simulink model "AxleSplitHEVv6"  (Simulink 8.5)
settings: Solver=ode5  StartTime=0.0  StopTime=hev_te  FixedStep=hev_dt  MaxStep=0.01  RelTol=1e-3  AbsTol=1e-3
PostLoadFcn:
  | load('AxelSplitHEVv4_NEDC_18_06_15.mat')
values from neighbouring files (symbols this model uses):
  cmd_equivalent_conso_coef = 0.11126984    [AxelSplitHEVv4_NEDC_18_06_15.mat]
  cmd_qmax = 42    [AxelSplitHEVv4_NEDC_18_06_15.mat]
  cmd_specific_volume_l_per_g = 0.00133333333333    [AxelSplitHEVv4_NEDC_18_06_15.mat]
  dri_cycle_speed_sp = [0 0 0 4.16666667 4.16666667 2.777777778 0 0 0 4.166666667 4.166666667 8.88888889 ... (135 elements, 135x1)]    [AxelSplitHEVv4_NEDC_18_06_15.mat]
  dri_cycle_speed_time = [0 6 11 15 23 25 28 44 49 54 56 61 ... (135 elements, 135x1)]    [AxelSplitHEVv4_NEDC_18_06_15.mat]
  dri_gbx_sp = [0 1 0 1 2 0 1 2 3 2 0 1 ... (52 elements, 52x1)]    [AxelSplitHEVv4_NEDC_18_06_15.mat]
  dri_gbx_time = [0 11 25 49 55 93 117 123 134 177 185 206 ... (52 elements, 52x1)]    [AxelSplitHEVv4_NEDC_18_06_15.mat]
  dri_ki = 24.5    [AxelSplitHEVv4_NEDC_18_06_15.mat]
  dri_kp = 609    [AxelSplitHEVv4_NEDC_18_06_15.mat]
  fa_clu_pos = [1 1 0.7 0.5 0.3 0 0]    [AxelSplitHEVv4_NEDC_18_06_15.mat]
  fa_clu_pv = [0 0.1 0.3 0.5 0.7 0.9 1]    [AxelSplitHEVv4_NEDC_18_06_15.mat]
  fa_conso_idle = 0.153611111111    [AxelSplitHEVv4_NEDC_18_06_15.mat]
  fa_conso_speed = [200 300 400 500 600 700 800 900 1000 1100 1200 1300 ... (56 elements, 1x56)]    [AxelSplitHEVv4_NEDC_18_06_15.mat]
  fa_conso_torque = [0 6.66666666667 13.3333333333 20 26.6666666667 33.3333333333 40 46.6666666667 53.3333333333 60 66.6666666667 73.3333333333 ... (43 elements, 1x43)]    [AxelSplitHEVv4_NEDC_18_06_15.mat]
  fa_delta_derating = 500    [AxelSplitHEVv4_NEDC_18_06_15.mat]
  fa_differential_ratio = FDR.fa_differential_ratio    [Algorithme_eff.m]    (also in AxelSplitHEVv4_NEDC_18_06_15.mat = 3.72; fa_differential_ratio.mat = 3.72)
  fa_fuel_consumption = [nan nan nan nan nan nan nan nan nan nan nan nan ... (2408 elements, 43x56)]    [AxelSplitHEVv4_NEDC_18_06_15.mat]    (also in Curve_fitting_conso.m = fa_fuel_consumption/max(max(fa_fuel_consumption)))
  fa_gearbox_efficiency = 0.92    [AxelSplitHEVv4_NEDC_18_06_15.mat]
  fa_gearbox_ratio = FGR.fa_gearbox_ratio    [Algorithme_eff.m]    (also in AxelSplitHEVv4_NEDC_18_06_15.mat = [0 3.98 2.21 1.47 1.1 0.89 0.75]; fa_gearbox_ratio.mat = [0 3.98 2.21 1.47 1.1 0.89 0.75])
  fa_high_derating_point = 5700    [AxelSplitHEVv4_NEDC_18_06_15.mat]
  fa_ice_inertia = 0.058    [AxelSplitHEVv4_NEDC_18_06_15.mat]
  fa_kp_idle_tr_off = 0.116198282851    [AxelSplitHEVv4_NEDC_18_06_15.mat]
  fa_kp_idle_tr_on = [1 0.8653 2.8063 6.3428 11.3274 17.3036 24.3665]    [AxelSplitHEVv4_NEDC_18_06_15.mat]
  fa_low_derating_point = 4000    [AxelSplitHEVv4_NEDC_18_06_15.mat]
  fa_max_tq_clu = 206    [AxelSplitHEVv4_NEDC_18_06_15.mat]
  fa_max_tq_ice = [0 220 233.333333333 240 246.666666667 253.333333333 253.333333333 253.333333333 260 260 266.666666667 266.666666667 ... (52 elements, 1x52)]    [AxelSplitHEVv4_NEDC_18_06_15.mat]
  fa_n_ice = [0 20 250 850 1000 1250 1500 1750 2000 2250 2500 3000 ... (18 elements, 1x18)]    [AxelSplitHEVv4_NEDC_18_06_15.mat]
  fa_starter_rpm = [0 10 20 30 40 50 60 70 80 90 100 110 ... (101 elements, 1x101)]    [AxelSplitHEVv4_NEDC_18_06_15.mat]
  fa_starter_tq = [24 24 24 24 23.3333333333 23.3333333333 23.3333333333 22.6666666667 22.6666666667 22 21.3333333333 20.6666666667 ... (101 elements, 1x101)]    [AxelSplitHEVv4_NEDC_18_06_15.mat]
  fa_tau_ice = 0.0333    [AxelSplitHEVv4_NEDC_18_06_15.mat]
  fa_taui_idle_tr_off = 0.0820482966067    [AxelSplitHEVv4_NEDC_18_06_15.mat]
  fa_taui_idle_tr_on = 0.194086623254    [AxelSplitHEVv4_NEDC_18_06_15.mat]
  fa_tq_loss = [0 -11 -10 -9 -9 -10 -11 -11 -12 -13 -14 -15 ... (18 elements, 1x18)]    [AxelSplitHEVv4_NEDC_18_06_15.mat]
  fa_tq_max_speed = [200 700 800 900 1000 1100 1200 1300 1400 1500 1600 1700 ... (52 elements, 1x52)]    [AxelSplitHEVv4_NEDC_18_06_15.mat]
  hev_dt = 0.01    [AxelSplitHEVv4_NEDC_18_06_15.mat]
  pla_csat = 1.2    [AxelSplitHEVv4_NEDC_18_06_15.mat]
  pla_equivalent_weight = 1250    [AxelSplitHEVv4_NEDC_18_06_15.mat]
  pla_f = 0.0035272    [AxelSplitHEVv4_NEDC_18_06_15.mat]
  pla_k = 0.0002318    [AxelSplitHEVv4_NEDC_18_06_15.mat]
  pla_kaero = 0.52992    [AxelSplitHEVv4_NEDC_18_06_15.mat]
  pla_max_f_brakes = 1000    [AxelSplitHEVv4_NEDC_18_06_15.mat]
  pla_wheel_radius = 0.314    [AxelSplitHEVv4_NEDC_18_06_15.mat]
  ra_differential_ratio = RDR.ra_differential_ratio    [Algorithme_eff.m]    (also in AxelSplitHEVv4_NEDC_18_06_15.mat = 10; ra_differential_ratio.mat = 10)
  ra_electrical_machine_efficiency = [nan nan nan nan nan nan nan 91.3 91.3 91.3 91.5 91.3 ... (777 elements, 37x21)]    [AxelSplitHEVv4_NEDC_18_06_15.mat]
  ra_electrical_machine_speed = [-12000 -10800 -9600 -8400 -7200 -6000 -4800 -3600 -2400 -1200 0 1200 ... (21 elements, 1x21)]    [AxelSplitHEVv4_NEDC_18_06_15.mat]
  ra_electrical_machine_tau = 0.1    [AxelSplitHEVv4_NEDC_18_06_15.mat]
  ra_electrical_machine_torque = [-79.6460176991 -75.2212389381 -70.796460177 -66.3716814159 -61.9469026549 -57.5221238938 -53.0973451327 -48.6725663717 -44.2477876106 -39.8230088496 -35.3982300885 -30.9734513274 ... (37 elements, 1x37)]    [AxelSplitHEVv4_NEDC_18_06_15.mat]
  ra_em_max_tq = [39.8230088496 44.2477876106 53.0973451327 57.5221238938 70.796460177 79.6460176991 79.6460176991 79.6460176991 79.6460176991 79.6460176991 79.6460176991 79.6460176991 ... (21 elements, 1x21)]    [AxelSplitHEVv4_NEDC_18_06_15.mat]
  ra_em_min_tq = [-39.8230088496 -44.2477876106 -53.0973451327 -57.5221238938 -70.796460177 -79.6460176991 -79.6460176991 -79.6460176991 -79.6460176991 -79.6460176991 -79.6460176991 -79.6460176991 ... (21 elements, 1x21)]    [AxelSplitHEVv4_NEDC_18_06_15.mat]
  ra_transmission_efficiency = 0.92    [AxelSplitHEVv4_NEDC_18_06_15.mat]
  syse_aux_current = 33.3    [AxelSplitHEVv4_NEDC_18_06_15.mat]
  syse_aux_voltage = 12    [AxelSplitHEVv4_NEDC_18_06_15.mat]
  syse_bat_nominal_capacity_as = 151200    [AxelSplitHEVv4_NEDC_18_06_15.mat]
  syse_cdl = 5000    [AxelSplitHEVv4_NEDC_18_06_15.mat]
  syse_dcdc_efficency = [78 89.6 92.5 95.2 95 94.6]    [AxelSplitHEVv4_NEDC_18_06_15.mat]
  syse_dcdc_in_power = [54 135 202 405 1485 2000]    [AxelSplitHEVv4_NEDC_18_06_15.mat]
  syse_electrical_machine_torque_vs_power_speed_nneg = [38.4209635438 42.3166718474 53.0973451327 53.8788373627 63.500986907 77.9700595469 78.3175021924 76.9635177026 72.2987813984 47.9837613501 38.4209635438 42.3166718474 ... (220 elements, 10x22)]    [AxelSplitHEVv4_NEDC_18_06_15.mat]
  syse_electrical_machine_torque_vs_power_speed_npos = [-72.2987813984 -76.9635177026 -78.3175021924 -77.9700595469 -63.500986907 -53.8788373627 -53.0973451327 -42.3166718474 -38.4209635438 -72.2987813984 -76.9635177026 -78.3175021924 ... (198 elements, 9x22)]    [AxelSplitHEVv4_NEDC_18_06_15.mat]
  syse_em_in_power = [-49.1089315336 -44.1089315336 -39.1089315336 -34.1089315336 -29.1089315336 -24.1089315336 -19.1089315336 -14.1089315336 -9.10893153364 -4.10893153364 0.891068466363 5.89106846636 ... (22 elements, 1x22)]    [AxelSplitHEVv4_NEDC_18_06_15.mat]
  syse_max_charge_current = [8.4 8.4 42 92.4 92.4 92.4 92.4 92.4 79.8 42 21 4.2]    [AxelSplitHEVv4_NEDC_18_06_15.mat]
  syse_max_discharge_current = [42 42 79.8 159.6 180.6 180.6 180.6 180.6 180.6 180.6 180.6 180.6]    [AxelSplitHEVv4_NEDC_18_06_15.mat]
  syse_nb_cell = 52    [AxelSplitHEVv4_NEDC_18_06_15.mat]
  syse_rdl = 0.004    [AxelSplitHEVv4_NEDC_18_06_15.mat]
  syse_rser = 0.002    [AxelSplitHEVv4_NEDC_18_06_15.mat]
  syse_soc_current_limits = [0 10 20 20.1 30 40 50 60 70 80 90 100]    [AxelSplitHEVv4_NEDC_18_06_15.mat]
  syse_soc_initial = 0.8    [AxelSplitHEVv4_NEDC_18_06_15.mat]
  syse_soc_ocv = [0 5 10 20 40 50 60 70 80 90 100]    [AxelSplitHEVv4_NEDC_18_06_15.mat]
  syse_vocv = [2.5 3.2135 3.5127 3.66 3.7771 3.8181 3.8686 3.8978 3.9429 4.0006 4.198]    [AxelSplitHEVv4_NEDC_18_06_15.mat]
libraries: simulink x20, simulink_extras x1
(part 2 of 3)

== system AxleSplitHEVv6/HEV model/Command/Braking_repartition/BREAKE REPARTITION RA ==
  CMD_RA_BREAK : Inport
  SYSE_SOC : Inport  Port=2
  RA_TQ_MIN : Inport  Port=3
  Add : Sum  Inputs=+-
  Add1 : Sum  Inputs=++|
  Add2 : Sum  Inputs=|+-
  Constant : Constant  Tag=Soc_level  Value=0.9
  Gain : Gain  Gain=-1
  Ground : Ground
  Switch : Switch  Criteria=u2 > Threshold
  Switch1 : Switch  Criteria=u2 > Threshold
  CMD_RA_MECHANICAL_BRAKE : Outport
  CMD_RA_ELECTRICAL_BRAKE : Outport  Port=2
  wires:
  CMD_RA_BREAK/1 -> Add1/1, Switch1/3, Add2/1
  Switch1/1 -> CMD_RA_ELECTRICAL_BRAKE/1, Add2/2
  Add1/1 -> Switch1/2
  Ground/1 -> Switch/1
  RA_TQ_MIN/1 -> Switch/3
  Switch/1 -> Gain/1, Add1/2
  Add2/1 -> CMD_RA_MECHANICAL_BRAKE/1
  SYSE_SOC/1 -> Add/1
  Constant/1 -> Add/2
  Add/1 -> Switch/2
  Gain/1 -> Switch1/1

== system AxleSplitHEVv6/HEV model/Command/Start_Stop/startstop prototype ==
  PLA_N : Inport
  DRI_GBX_SP : Inport  Port=2
  START_STOP_ENABLE : Inport  Port=3
  DRI_CLUTCH_SP : Inport  Port=4
  Activate Start/Stopo strategy : Constant  Value=0
  Logical Operator1 : Logic  Inputs=3  AllPortsSameDT=off  OutDataTypeStr=boolean  SampleTime=hev_dt
  Switch : Switch  Criteria=u2 ~= 0  SampleTime=hev_dt
  car_moving : simulink/Logic and Bit Operations/Compare To Constant  relop=<=  const=0.04  OutDataTypeStr=uint8
  clutch_pedal_down : simulink/Logic and Bit Operations/Compare To Constant  relop===  const=1  OutDataTypeStr=uint8
  gbx_not_neutral : simulink/Logic and Bit Operations/Compare To Constant  relop===  const=0  OutDataTypeStr=uint8
  CMD_ICE_ENABLE : Outport
  wires:
  PLA_N/1 -> car_moving/1
  car_moving/1 -> Logical Operator1/1
  gbx_not_neutral/1 -> Logical Operator1/3
  Activate Start/Stopo strategy/1 -> Switch/3
  Logical Operator1/1 -> Switch/1
  DRI_GBX_SP/1 -> gbx_not_neutral/1
  START_STOP_ENABLE/1 -> Switch/2
  Switch/1 -> CMD_ICE_ENABLE/1
  DRI_CLUTCH_SP/1 -> clutch_pedal_down/1
  clutch_pedal_down/1 -> Logical Operator1/2

== system AxleSplitHEVv6/HEV model/Command/Torque repartition/Optimization Algorithm  ==
  note: Filtrage du alpha
  T : Inport
  PLA_N : Inport  Port=2
  Tmax_elec : Inport  Port=3
  Tmin_elec : Inport  Port=4
  Tmax_therm : Inport  Port=5
  Tmin_therm : Inport  Port=6
  DRI_GBX : Inport  Port=7
  "SOC " : Inport  Port=8
  Doc Front axle : Subsystem
      settings: OpenFcn=open('Documents\Command Torque Repartition Algorithm.pdf')
      mask Display: fprintf('DOC')
  Doc Front axle1 : Subsystem
      settings: OpenFcn=open('Optimization_Algorithm')
      mask Display: fprintf('Generate\nOptimization\nAlgorithm\nSfunction')
  Sfunction: Optimization Algorithm 32bits : Subsystem
      mask help: Simulink:masks:GenSFuncDesc_MD
      mask Help: eval('feval(''rtwprivate'',''rtwhelpview'',''rtw_sfcn_block'')');
  Transfer Fcn : TransferFcn  Denominator=[1 3/2]
  alpha : Outport
  wires:
  Tmax_elec/1 -> Sfunction: Optimization Algorithm 32bits/3(Tmax_elec)
  Tmin_elec/1 -> Sfunction: Optimization Algorithm 32bits/4(Tmin_elec)
  PLA_N/1 -> Sfunction: Optimization Algorithm 32bits/2(V)
  Tmax_therm/1 -> Sfunction: Optimization Algorithm 32bits/5(Tmax_therm)
  T/1 -> Sfunction: Optimization Algorithm 32bits/1(T)
  Tmin_therm/1 -> Sfunction: Optimization Algorithm 32bits/6(Tmin_therm)
  DRI_GBX/1 -> Sfunction: Optimization Algorithm 32bits/7(GBX)
  "SOC "/1 -> Sfunction: Optimization Algorithm 32bits/8(SOC)
  Transfer Fcn/1 -> alpha/1
  Sfunction: Optimization Algorithm 32bits/1(alpha_opt) -> Transfer Fcn/1

== system AxleSplitHEVv6/HEV model/Command/Torque repartition/energy_manager Stop thermal engine when <20km/h ==
  note: Energy managment modified : Not taking account of the FA_START command
      | Cf. Previous model
  PLA_N : Inport
  alpha_in : Inport  Port=2
  SOC : Inport  Port=3
  Compare To Constant : simulink/Logic and Bit Operations/Compare To Constant  relop=<  const=20  OutDataTypeStr=boolean
  Compare To Constant1 : simulink/Logic and Bit Operations/Compare To Constant  relop=>  const=0.2  OutDataTypeStr=boolean
  Constant3 : Constant  Value=0
  Gain : Gain  Gain=(60*(2*pi*pla_wheel_radius))/1e3
  Logical Operator1 : Logic  AllPortsSameDT=off  OutDataTypeStr=boolean
  Switch : Switch  Criteria=u2 > Threshold
  alpha_out : Outport
  CMD_ENERGY_MANAGER : Outport  Port=2
  wires:
  SOC/1 -> Compare To Constant1/1
  PLA_N/1 -> Gain/1
  Logical Operator1/1 -> CMD_ENERGY_MANAGER/1, Switch/2
  Compare To Constant1/1 -> Logical Operator1/1
  Gain/1 -> Compare To Constant/1
  Constant3/1 -> Switch/1
  alpha_in/1 -> Switch/3
  Switch/1 -> alpha_out/1
  Compare To Constant/1 -> Logical Operator1/2

== system AxleSplitHEVv6/HEV model/Driver1/Clutch command/Clutch Command ==
  note: SHIFT DOWN
  note: SHIFT UP
  DRI_REF_GBX : Inport
  Data Type Conversion : DataTypeConversion  OutDataTypeStr=double
  Data Type Conversion1 : DataTypeConversion  OutDataTypeStr=double
  Delay : Delay  DelayLength=1/hev_dt
  Delay1 : Delay  DelayLength=1
  Delay2 : Delay  DelayLength=1
  SHIFT DOWN : Stateflow chart  TreatAsAtomicUnit=on
  SHIFT UP : Stateflow chart  TreatAsAtomicUnit=on
  Sum2 : Sum
  To Workspace : ToWorkspace  VariableName=GBX_reference  SampleTime=-1
  Transfer Fcn{1..4} (4 alike) : TransferFcn  Denominator=[0.1 1]
  DRI_CLUTCH_SP : Outport
  DRI_GBX_SP : Outport  Port=2
  wires:
  SHIFT UP/1(output_memory) -> Data Type Conversion/1
  Sum2/1 -> DRI_CLUTCH_SP/1
  SHIFT DOWN/1(output_memory) -> Data Type Conversion1/1
  Delay2/1 -> SHIFT DOWN/1(last_DRI_REF_GBX)
  DRI_REF_GBX/1 -> SHIFT UP/2(DRI_REF_GBX), Delay1/1, Delay/1, SHIFT DOWN/2(DRI_REF_GBX), Delay2/1, To Workspace/1
  Delay/1 -> SHIFT UP/3(actual_DRI_GBX), DRI_GBX_SP/1, SHIFT DOWN/3(actual_DRI_GBX)
  Delay1/1 -> SHIFT UP/1(last_DRI_REF_GBX)
  Transfer Fcn1/1 -> Transfer Fcn2/1
  Data Type Conversion/1 -> Transfer Fcn1/1
  Transfer Fcn3/1 -> Transfer Fcn4/1
  Data Type Conversion1/1 -> Transfer Fcn3/1
  Transfer Fcn2/1 -> Sum2/1
  Transfer Fcn4/1 -> Sum2/2

== system AxleSplitHEVv6/HEV model/Driver1/Clutch command/Clutch Stuck ==
  REF_GBX : Inport
  FA_N_ICE : Inport  Port=2
  DRI_CLU_SP : Inport  Port=3
  1/time pedal down->up  gbx 1st gear : Constant  Value=-1/2
  1/time pedal up->down : Constant  Value=2
  Compare To Constant : simulink/Logic and Bit Operations/Compare To Constant  relop=>=  const=2000  OutDataTypeStr=boolean
  Compare To Constant1 : simulink/Logic and Bit Operations/Compare To Constant  relop=<  const=800  OutDataTypeStr=boolean
  Compare To Constant3 : simulink/Logic and Bit Operations/Compare To Constant  relop===  const=0  OutDataTypeStr=uint8
  Compare To Constant4 : simulink/Logic and Bit Operations/Compare To Constant  relop=~=  const=0  OutDataTypeStr=uint8
  Data Type Conversion4 : DataTypeConversion  OutDataTypeStr=double  SampleTime=hev_dt
  Delay1 : Delay  DelayLength=2/hev_dt  SampleTime=hev_dt
  Delay2 : Delay  DelayLength=1  SampleTime=hev_dt
  Logical Operator1 : Logic  Operator=OR  AllPortsSameDT=off  OutDataTypeStr=boolean  SampleTime=hev_dt
  Logical Operator7 : Logic  Inputs=3  AllPortsSameDT=off  OutDataTypeStr=boolean  SampleTime=hev_dt
  Rate Limiter Dynamic : simulink/Discontinuities/Rate Limiter Dynamic
  S-R Flip-Flop : simulink_extras/Flip Flops/S-R Flip-Flop  initial_condition=0
  Switch : Switch  Criteria=u2 > Threshold
  Terminator : Terminator
  OUT_CLU : Outport
  wires:
  REF_GBX/1 -> Delay2/1, Compare To Constant4/1
  S-R Flip-Flop/2 -> Terminator/1
  Compare To Constant/1 -> S-R Flip-Flop/2
  Rate Limiter Dynamic/1 -> Switch/1
  S-R Flip-Flop/1 -> Logical Operator1/2, Delay1/1, Data Type Conversion4/1
  Compare To Constant4/1 -> Logical Operator7/1
  Delay2/1 -> Compare To Constant3/1
  Compare To Constant3/1 -> Logical Operator7/2
  FA_N_ICE/1 -> Compare To Constant/1, Compare To Constant1/1
  Delay1/1 -> Logical Operator1/1
  Data Type Conversion4/1 -> Rate Limiter Dynamic/2
  1/time pedal up->down/1 -> Rate Limiter Dynamic/1
  Compare To Constant1/1 -> Logical Operator7/3
  Logical Operator1/1 -> Switch/2
  Logical Operator7/1 -> S-R Flip-Flop/1
  1/time pedal down->up  gbx 1st gear/1 -> Rate Limiter Dynamic/3
  Switch/1 -> OUT_CLU/1
  DRI_CLU_SP/1 -> Switch/3

== system AxleSplitHEVv6/HEV model/Electrical system/Auxiliary network 12V/Auxliliary network ==
  Constant : Constant  Value=syse_aux_current
  Constant1 : Constant  Value=syse_aux_voltage
  SYSE_CURRENT_LV : Outport
  SYSE_VOLTAGE_LV : Outport  Port=2
  wires:
  Constant/1 -> SYSE_CURRENT_LV/1  "A"
  Constant1/1 -> SYSE_VOLTAGE_LV/1  "V"

== system AxleSplitHEVv6/HEV model/Electrical system/Auxiliary network 12V/CVS ==
  note: V
  SYSE_CURRENT_LV : Inport
  SYSE_VOLTAGE_LV : Inport  Port=2
  SYSE_VOLTAGE_HV : Inport  Port=3
  Delay : Delay  DelayLength=1  SampleTime=hev_dt
  Divide : Product  Inputs=/*  SampleTime=hev_dt
  Divide1 : Product  Inputs=*/  SampleTime=hev_dt
  Product : Product  SampleTime=hev_dt  RndMeth=Zero
  rendement CVS : Lookup_n-D  NumberOfTableDimensions=1  BreakpointsForDimension1=syse_dcdc_in_power.*(syse_dcdc_efficency/100)  Table=syse_dcdc_efficency/100  SampleTime=hev_dt  RndMeth=Simplest  InputSameDT=on
  SYSE_AUX_CURRENT : Outport
  wires:
  rendement CVS/1 -> Divide/1
  Divide/1 -> Divide1/1  "W"
  Product/1 -> Divide/2, rendement CVS/1  "W"
  SYSE_VOLTAGE_HV/1 -> Divide1/2
  SYSE_CURRENT_LV/1 -> Product/1
  SYSE_VOLTAGE_LV/1 -> Product/2
  Divide1/1 -> Delay/1
  Delay/1 -> SYSE_AUX_CURRENT/1

== system AxleSplitHEVv6/HEV model/Electrical system/Electrical System supervision/Battery charge / discharge limits ==
  SYSE_SOC : Inport
  Courant Charge Lookup Table : Lookup_n-D  NumberOfTableDimensions=1  BreakpointsForDimension1=syse_soc_current_limits/100  Table=-syse_max_charge_current  SampleTime=hev_dt  RndMeth=Simplest  InputSameDT=on
  Courant Decharge Lookup Table : Lookup_n-D  NumberOfTableDimensions=1  BreakpointsForDimension1=syse_soc_current_limits/100  Table=syse_max_discharge_current  SampleTime=hev_dt  RndMeth=Simplest  InputSameDT=on
  SYSE_I_DISCHARGE : Outport
  SYSE_I_CHARGE : Outport  Port=2
  wires:
  SYSE_SOC/1 -> Courant Decharge Lookup Table/1, Courant Charge Lookup Table/1
  Courant Decharge Lookup Table/1 -> SYSE_I_DISCHARGE/1
  Courant Charge Lookup Table/1 -> SYSE_I_CHARGE/1

== system AxleSplitHEVv6/HEV model/Electrical system/Electrical System supervision/Current loop ==
  SYSE_AUX_CURRENT : Inport
  SYSE_I_DISCHARGE : Inport  Port=2
  SYSE_I_CHARGE : Inport  Port=3
  Subtract2 : Sum  Inputs=-+  SampleTime=hev_dt
  Subtract3 : Sum  SampleTime=hev_dt
  SYSE_EM_I_DISCHARGE : Outport
  SYSE_EM_I_CHARGE : Outport  Port=2
  wires:
  SYSE_AUX_CURRENT/1 -> Subtract2/1, Subtract3/1  "A"
  Subtract2/1 -> SYSE_EM_I_DISCHARGE/1  "A"
  SYSE_I_DISCHARGE/1 -> Subtract2/2  "A"
  Subtract3/1 -> SYSE_EM_I_CHARGE/1  "A"
  SYSE_I_CHARGE/1 -> Subtract3/2  "A"

== system AxleSplitHEVv6/HEV model/Electrical system/Electrical System supervision/Min max  ==
  note: RPM
  SYSE_EM_I_DISCHARGE : Inport
  SYSE_EM_I_CHARGE : Inport  Port=2
  SYSE_VOLTAGE_HV : Inport  Port=3
  PLA_N_EM : Inport  Port=4
  Min /w power neg : Lookup_n-D  BreakpointsForDimension1=ra_electrical_machine_speed(1:10)  BreakpointsForDimension2=syse_em_in_power*1000  Table=syse_electrical_machine_torque_vs_power_speed_nneg  ExtrapMethod=Clip  UseLastTableValue=on  SampleTime=hev_dt  RndMeth=Simplest  InputSameDT=on
  Min /w power pos : Lookup_n-D  BreakpointsForDimension1=ra_electrical_machine_speed(12:20)  BreakpointsForDimension2=syse_em_in_power*1000  Table=syse_electrical_machine_torque_vs_power_speed_npos  ExtrapMethod=Clip  UseLastTableValue=on  SampleTime=hev_dt  RndMeth=Simplest  InputSameDT=on
  Product : Product  SampleTime=hev_dt  RndMeth=Zero
  Product2 : Product  SampleTime=hev_dt  RndMeth=Zero
  Switch : Switch  Threshold=-5  SampleTime=hev_dt
  Switch1 : Switch  Threshold=-5  SampleTime=hev_dt
  max /w power neg : Lookup_n-D  BreakpointsForDimension1=ra_electrical_machine_speed(1:10)  BreakpointsForDimension2=syse_em_in_power*1000  Table=syse_electrical_machine_torque_vs_power_speed_nneg  ExtrapMethod=Clip  UseLastTableValue=on  SampleTime=hev_dt  RndMeth=Simplest  InputSameDT=on
  max /w power pos : Lookup_n-D  BreakpointsForDimension1=ra_electrical_machine_speed(12:20)  BreakpointsForDimension2=syse_em_in_power*1000  Table=syse_electrical_machine_torque_vs_power_speed_npos  ExtrapMethod=Clip  UseLastTableValue=on  SampleTime=hev_dt  RndMeth=Simplest  InputSameDT=on
  SYSE_TQ_MAX_BMS : Outport
  SYSE_TQ_MIN_BMS : Outport  Port=2
  wires:
  PLA_N_EM/1 -> Min /w power pos/1, Min /w power neg/1, Switch1/2, max /w power pos/1, max /w power neg/1, Switch/2
  SYSE_EM_I_DISCHARGE/1 -> Product/1  "A"
  SYSE_EM_I_CHARGE/1 -> Product2/1  "A"
  Product2/1 -> Min /w power pos/2, Min /w power neg/2  "W"
  Product/1 -> max /w power neg/2, max /w power pos/2  "W"
  SYSE_VOLTAGE_HV/1 -> Product2/2, Product/2
  Switch/1 -> SYSE_TQ_MAX_BMS/1
  max /w power pos/1 -> Switch/1
  max /w power neg/1 -> Switch/3  "Nm"
  Min /w power pos/1 -> Switch1/1  "Nm"
  Min /w power neg/1 -> Switch1/3
  Switch1/1 -> SYSE_TQ_MIN_BMS/1

== system AxleSplitHEVv6/HEV model/Electrical system/Electrical System supervision/Torque conversion ==
  SYSE_TQ_MINMAX_BMS : Inport
  RA_N_EM : Inport  Port=2
  Differential ratio : Gain  Gain=ra_differential_ratio  SampleTime=hev_dt
  Divide1 : Product  SampleTime=hev_dt
  Efficiency P neg : Gain  Gain=2-ra_transmission_efficiency  SampleTime=hev_dt
  Efficiency P pos : Gain  Gain=ra_transmission_efficiency  SampleTime=hev_dt
  Switch : Switch  SampleTime=hev_dt
  SYSE_TQ_MINMAX : Outport
  wires:
  SYSE_TQ_MINMAX_BMS/1 -> Divide1/2, Efficiency P neg/1, Efficiency P pos/1
  Efficiency P pos/1 -> Switch/1
  Efficiency P neg/1 -> Switch/3
  Divide1/1 -> Switch/2
  Switch/1 -> Differential ratio/1
  RA_N_EM/1 -> Divide1/1
  Differential ratio/1 -> SYSE_TQ_MINMAX/1

== system AxleSplitHEVv6/HEV model/Electrical system/Lithium-Ion Battery Management System/Battery control ==
  note: Battery safety system
  SYSE_LIION_CURRENT : Inport
  SYSE_SOC : Inport  Port=2
  Courant Charge Lookup Table : Lookup_n-D  NumberOfTableDimensions=1  BreakpointsForDimension1=syse_soc_current_limits/100  Table=-syse_max_charge_current  SampleTime=hev_dt  RndMeth=Simplest  InputSameDT=on
  Courant Decharge Lookup Table : Lookup_n-D  NumberOfTableDimensions=1  BreakpointsForDimension1=syse_soc_current_limits/100  Table=syse_max_discharge_current  SampleTime=hev_dt  RndMeth=Simplest  InputSameDT=on
  Logical Operator : Logic  AllPortsSameDT=off  OutDataTypeStr=boolean  SampleTime=hev_dt
  Relational Operator : RelationalOperator  Operator=<  OutDataTypeStr=boolean  SampleTime=hev_dt
  Relational Operator1 : RelationalOperator  Operator=>  OutDataTypeStr=boolean  SampleTime=hev_dt
  SYSE_LIION_CONTACTOR_OPEN_REQ : Outport
  wires:
  SYSE_LIION_CURRENT/1 -> Relational Operator/1, Relational Operator1/1  "A"
  Courant Charge Lookup Table/1 -> Relational Operator/2  "syse_max_charge_current (A)"
  Courant Decharge Lookup Table/1 -> Relational Operator1/2  "syse_max_discharge_current (A)"
  SYSE_SOC/1 -> Courant Charge Lookup Table/1, Courant Decharge Lookup Table/1
  Logical Operator/1 -> SYSE_LIION_CONTACTOR_OPEN_REQ/1
  Relational Operator/1 -> Logical Operator/1
  Relational Operator1/1 -> Logical Operator/2

== system AxleSplitHEVv6/HEV model/Electrical system/Lithium-Ion Battery Management System/Battery model ==
  SYSE_LIION_CURRENT_OUT : Inport
  li-ion Battery SOC : Subsystem
  li-ion battery voltage : Subsystem
  SYSE_VOLTAGE_HV : Outport
  SYSE_SOC : Outport  Port=2
  wires:
  li-ion battery voltage/1(SYSE_VOLTAGE_HV) -> SYSE_VOLTAGE_HV/1  "V"
  SYSE_LIION_CURRENT_OUT/1 -> li-ion Battery SOC/1(SYSE_LIION_CURRENT), li-ion battery voltage/2(SYSE_LIION_CURRENT)
  li-ion Battery SOC/1(SYSE_SOC) -> li-ion battery voltage/1(SYSE_SOC), SYSE_SOC/1

== system AxleSplitHEVv6/HEV model/Electrical system/Lithium-Ion Battery Management System/Battery power contactor ==
  SYSE_LIION_CONTACTOR_OPEN_REQ : Inport
  SYSE_LIION_CURRENT : Inport  Port=2
  Contactor : Switch  Criteria=u2 ~= 0  SampleTime=hev_dt
  OPEN : Constant  Value=0
  SYSE_LIION_CURRENT_OUT : Outport
  wires:
  OPEN/1 -> Contactor/1
  SYSE_LIION_CURRENT/1 -> Contactor/3
  SYSE_LIION_CONTACTOR_OPEN_REQ/1 -> Contactor/2
  Contactor/1 -> SYSE_LIION_CURRENT_OUT/1

== system AxleSplitHEVv6/HEV model/Front Axle/Clutch/Stuck logic ==
  FA_W_CAR_INTEGRATOR_STATE : Inport
  FA_W_CAR : Inport  Port=2
  FA_TQ_ICE : Inport  Port=3
  FA_CLU_MAX_STATIC_TORQUE : Inport  Port=4
  Abs : Abs  SampleTime=hev_dt  SaturateOnIntegerOverflow=on
  Abs1 : Abs  SampleTime=hev_dt  SaturateOnIntegerOverflow=on
  Abs2 : Abs  SampleTime=hev_dt  SaturateOnIntegerOverflow=on
  Combinatorial  Logic3 : CombinatorialLogic  Description=TRUTH_TABLE_FROM_FABIEN  TruthTable=[0;1;0;0;1;1;0;1]  SampleTime=hev_dt
  Compare To Constant : simulink/Logic and Bit Operations/Compare To Constant  relop=<=  const=40  OutDataTypeStr=boolean
  Delay : Delay  DelayLength=1  SampleTime=hev_dt
  Logic : Logic  IconShape=distinctive  SampleTime=hev_dt
  Mux : Mux  Inputs=3
  Relational Operator : RelationalOperator  Operator=<=  SampleTime=hev_dt  InputSameDT=on
  Relational Operator1 : RelationalOperator  Operator=<=  SampleTime=hev_dt  InputSameDT=on
  Scope2 : Scope
      settings: YMin=-1.5e-14  YMax=1.5e-14  SaveName=ScopeData14
  Sum1 : Sum  Inputs=+-  SampleTime=hev_dt  SaturateOnIntegerOverflow=on  InputSameDT=on  OutDataTypeStr=Inherit: Same as first input
  FA_CLU_STUCK : Outport
  wires:
  FA_CLU_MAX_STATIC_TORQUE/1 -> Relational Operator1/2, Relational Operator/1
  Sum1/1 -> Abs2/1
  Abs1/1 -> Relational Operator1/1
  Delay/1 -> Mux/3
  Combinatorial  Logic3/1 -> Delay/1, FA_CLU_STUCK/1
  Mux/1 -> Combinatorial  Logic3/1
  Abs/1 -> Relational Operator/2
  Relational Operator/1 -> Mux/2
  Logic/1 -> Mux/1
  Abs2/1 -> Compare To Constant/1
  Compare To Constant/1 -> Logic/1
  Relational Operator1/1 -> Scope2/1, Logic/2
  FA_TQ_ICE/1 -> Abs1/1, Abs/1
  FA_W_CAR_INTEGRATOR_STATE/1 -> Sum1/1
  FA_W_CAR/1 -> Sum1/2

== system AxleSplitHEVv6/HEV model/Front Axle/ICE/ICE ==
  FA_N_ICE : Inport
  FA_ICE_TQ_SP : Inport  Port=2
  FA_STARTER_REQUEST : Inport  Port=3
  FA_ICE_STATE : Inport  Port=4
  Add1 : Sum  Inputs=3  SampleTime=hev_dt
  Constant4 : Constant  Value=0
  Discrete Transfer Fcn3 : DiscreteTransferFcn  Numerator=[(hev_dt/(2*(fa_tau_ice)+hev_dt)) (hev_dt/(2*(fa_tau_ice)+hev_dt))]  Denominator=[1 ((hev_dt-2*(fa_tau_ice)))/(2*(fa_tau_ice)+hev_dt)]  SampleTime=hev_dt
  Gas consumption : Subsystem
  Switch1 : Switch  Criteria=u2 ~= 0  SampleTime=hev_dt
  TQ_LOSS : Lookup_n-D  NumberOfTableDimensions=1  BreakpointsForDimension1=fa_n_ice  Table=fa_tq_loss  UseLastTableValue=on  SampleTime=hev_dt  RndMeth=Simplest  InputSameDT=on
  TQ_STARTER : Lookup_n-D  NumberOfTableDimensions=1  BreakpointsForDimension1=fa_starter_rpm  Table=fa_starter_tq  ExtrapMethod=Clip  UseLastTableValue=on  SampleTime=hev_dt  RndMeth=Simplest  InputSameDT=on
  FA_GAS_CONSUMPTION : Outport
  FA_TQ_ICE : Outport  Port=2
  FA_TQ_STARTER : Outport  Port=3
  wires:
  TQ_LOSS/1 -> Add1/3
  Discrete Transfer Fcn3/1 -> Gas consumption/2(FA_TQ_ICE_OFFSET), Add1/1
  Constant4/1 -> Switch1/3
  Switch1/1 -> Add1/2, FA_TQ_STARTER/1
  FA_N_ICE/1 -> Gas consumption/1(FA_N_ICE), TQ_LOSS/1, TQ_STARTER/1
  Gas consumption/1(FA_GAS_CONSUMPTION) -> FA_GAS_CONSUMPTION/1
  FA_ICE_TQ_SP/1 -> Discrete Transfer Fcn3/1
  Add1/1 -> FA_TQ_ICE/1
  FA_STARTER_REQUEST/1 -> Switch1/2
  TQ_STARTER/1 -> Switch1/1
  FA_ICE_STATE/1 -> Gas consumption/3(FA_ICE_STATE)

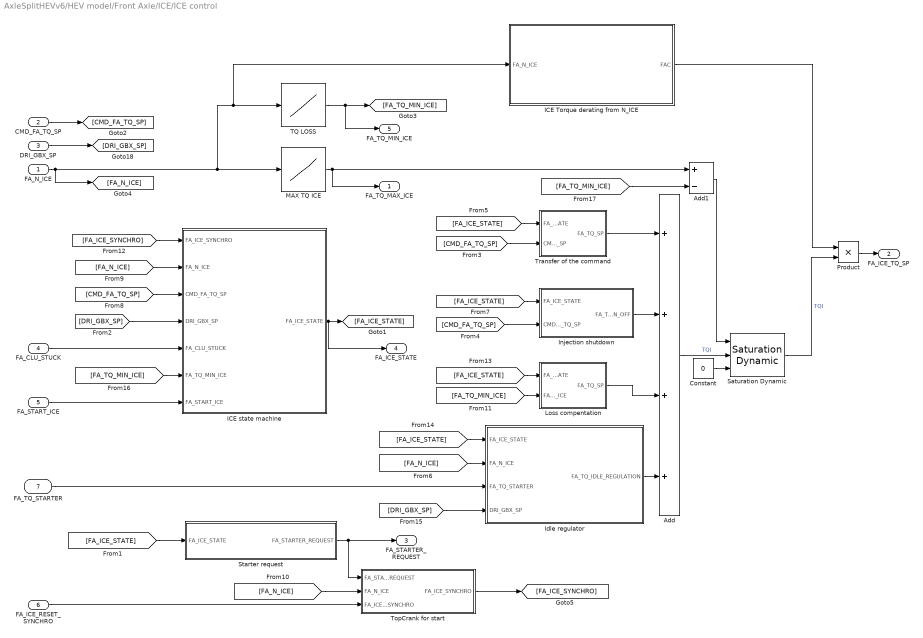
== system AxleSplitHEVv6/HEV model/Front Axle/ICE/ICE control ==
  FA_N_ICE : Inport
  CMD_FA_TQ_SP : Inport  Port=2
  DRI_GBX_SP : Inport  Port=3
  FA_CLU_STUCK : Inport  Port=4
  FA_START_ICE : Inport  Port=5
  FA_ICE_RESET_SYNCHRO : Inport  Port=6
  FA_TQ_STARTER : Inport  Port=7
  Add : Sum  Inputs=4  SampleTime=hev_dt
  Add1 : Sum  Inputs=+-  SampleTime=hev_dt
  Constant : Constant  Value=0
  ICE Torque derating from N_ICE : Subsystem
  ICE state machine : Stateflow chart  TreatAsAtomicUnit=on
  Idle regulator : Subsystem
  Injection shutdown : Subsystem
  Loss compentation : Subsystem
  MAX TQ ICE : Lookup_n-D  NumberOfTableDimensions=1  BreakpointsForDimension1=fa_tq_max_speed  Table=fa_max_tq_ice  ExtrapMethod=Clip  UseLastTableValue=on  SampleTime=hev_dt  RndMeth=Simplest  InputSameDT=on
  Product : Product
  Saturation Dynamic : simulink/Discontinuities/Saturation Dynamic  OutMin=[]  OutMax=[]  OutDataTypeStr=Inherit: Same as second input  OutDataType=fixdt(1, 16)  OutScaling=2^-10  DoSatur=off
  Starter request : Subsystem
  TQ LOSS : Lookup_n-D  NumberOfTableDimensions=1  BreakpointsForDimension1=fa_n_ice  Table=fa_tq_loss  UseLastTableValue=on  SampleTime=hev_dt  RndMeth=Simplest  InputSameDT=on
  TopCrank for start : Subsystem
  Transfer of the command : Subsystem
  FA_TQ_MAX_ICE : Outport
  FA_ICE_TQ_SP : Outport  Port=2
  FA_STARTER_REQUEST : Outport  Port=3
  FA_ICE_STATE : Outport  Port=4
  FA_TQ_MIN_ICE : Outport  Port=5
  wires:
  DRI_GBX_SP/1 -> [DRI_GBX_SP]
  [DRI_GBX_SP] -> ICE state machine/4(DRI_GBX_SP)
  ICE state machine/1(FA_ICE_STATE) -> [FA_ICE_STATE], FA_ICE_STATE/1
  Injection shutdown/1(FA_TQ_SP_INJECTION_OFF) -> Add/2
  Transfer of the command/1(FA_TQ_SP) -> Add/1
  [FA_ICE_STATE] -> Transfer of the command/1(FA_ICE_STATE)
  [CMD_FA_TQ_SP] -> Injection shutdown/2(CMD_FA_TQ_SP)
  Starter request/1(FA_STARTER_REQUEST) -> TopCrank for start/1(FA_STARTER_REQUEST), FA_STARTER_REQUEST/1
  [FA_ICE_STATE] -> Starter request/1(FA_ICE_STATE)
  Add/1 -> Saturation Dynamic/2  "TQI"
  MAX TQ ICE/1 -> FA_TQ_MAX_ICE/1, Add1/1
  CMD_FA_TQ_SP/1 -> [CMD_FA_TQ_SP]
  [CMD_FA_TQ_SP] -> ICE state machine/3(CMD_FA_TQ_SP)
  FA_N_ICE/1 -> [FA_N_ICE], MAX TQ ICE/1, ICE Torque derating from N_ICE/1(FA_N_ICE), TQ LOSS/1
  [FA_ICE_STATE] -> Injection shutdown/1(FA_ICE_STATE)
  FA_CLU_STUCK/1 -> ICE state machine/5(FA_CLU_STUCK)
  [FA_ICE_SYNCHRO] -> ICE state machine/1(FA_ICE_SYNCHRO)
  [FA_ICE_STATE] -> Loss compentation/1(FA_ICE_STATE)
  TopCrank for start/1(FA_ICE_SYNCHRO) -> [FA_ICE_SYNCHRO]
  Constant/1 -> Saturation Dynamic/3
  Add1/1 -> Saturation Dynamic/1
  FA_ICE_RESET_SYNCHRO/1 -> TopCrank for start/3(FA_ICE_RESET_SYNCHRO)
  FA_START_ICE/1 -> ICE state machine/7(FA_START_ICE)
  Saturation Dynamic/1 -> Product/2  "TQI"
  Loss compentation/1(FA_TQ_SP) -> Add/3
  [FA_ICE_STATE] -> Idle regulator/1(FA_ICE_STATE)
  [DRI_GBX_SP] -> Idle regulator/4(DRI_GBX_SP)
  Idle regulator/1(FA_TQ_IDLE_REGULATION) -> Add/4
  FA_TQ_STARTER/1 -> Idle regulator/3(FA_TQ_STARTER)
  [FA_N_ICE] -> Idle regulator/2(FA_N_ICE)
  [FA_N_ICE] -> ICE state machine/2(FA_N_ICE)
  TQ LOSS/1 -> FA_TQ_MIN_ICE/1, [FA_TQ_MIN_ICE]
  [FA_N_ICE] -> TopCrank for start/2(FA_N_ICE)
  [FA_TQ_MIN_ICE] -> Loss compentation/2(FA_TQ_MIN_ICE)
  [FA_TQ_MIN_ICE] -> ICE state machine/6(FA_TQ_MIN_ICE)
  [FA_TQ_MIN_ICE] -> Add1/2
  [CMD_FA_TQ_SP] -> Transfer of the command/2(CMD_FA_TQ_SP)
  ICE Torque derating from N_ICE/1(FAC) -> Product/1
  Product/1 -> FA_ICE_TQ_SP/1

== system AxleSplitHEVv6/HEV model/Platform/Mechanical behavior/Adherence ==
  PLA_SUM_FORCES_OVER_EQ_WEIGHT : Inport
  PLA_SUM_FORCES : Inport  Port=2
  PLA_SPEED_MS : Inport  Port=3
  Abs : Abs  SampleTime=hev_dt
  Abs1 : Abs  SampleTime=hev_dt
  Compare To Constant : simulink/Logic and Bit Operations/Compare To Constant  relop=<=  const=0.01  OutDataTypeStr=uint8
  Compare To Constant1 : simulink/Logic and Bit Operations/Compare To Constant  relop=<=  const=9.80665*pla_equivalent_weight*pla_f*pla_csat  OutDataTypeStr=uint8
  Constant : Constant  Value=0
  Logical Operator : Logic  AllPortsSameDT=off  OutDataTypeStr=boolean  SampleTime=hev_dt
  Switch : Switch  Criteria=u2 ~= 0  SampleTime=hev_dt
  PLA_SUM_TO_INTEGRATOR : Outport
  wires:
  PLA_SUM_FORCES_OVER_EQ_WEIGHT/1 -> Switch/3
  Switch/1 -> PLA_SUM_TO_INTEGRATOR/1
  PLA_SPEED_MS/1 -> Abs/1
  PLA_SUM_FORCES/1 -> Abs1/1
  Abs1/1 -> Compare To Constant1/1
  Abs/1 -> Compare To Constant/1
  Constant/1 -> Switch/1
  Compare To Constant1/1 -> Logical Operator/2
  Logical Operator/1 -> Switch/2
  Compare To Constant/1 -> Logical Operator/1

== system AxleSplitHEVv6/HEV model/Platform/Mechanical behavior/Faero ==
  PLA_SPEED_MS : Inport
  ENV_WIND_SPEED : Inport  Port=2
  Gain : Gain  Gain=-1  SampleTime=hev_dt
  Gain1 : Gain  Gain=pla_kaero  SampleTime=hev_dt
  Product : Product  SampleTime=hev_dt
  Product1 : Product  SampleTime=hev_dt
  Sign : Signum  SampleTime=hev_dt
  Sum : Sum  Inputs=+|+  SampleTime=hev_dt
  PLA_FORCE_AERO : Outport
  wires:
  PLA_SPEED_MS/1 -> Sign/1, Sum/1
  ENV_WIND_SPEED/1 -> Sum/2
  Sum/1 -> Product/2, Product/1
  Product/1 -> Gain1/1
  Gain1/1 -> Product1/2
  Product1/1 -> Gain/1
  Sign/1 -> Product1/1
  Gain/1 -> PLA_FORCE_AERO/1

== system AxleSplitHEVv6/HEV model/Platform/Mechanical behavior/Fbrakes ==
  CMD_BRAKE_SP : Inport
  PLA_SPEED_MS : Inport  Port=2
  Gain2 : Gain  Gain=-1  SampleTime=hev_dt
  Product1 : Product  SampleTime=hev_dt
  Saturation : Saturate  UpperLimit=pla_max_f_brakes  LowerLimit=0
  Sign : Signum  SampleTime=hev_dt
  PLA_FORCE_BRAKE : Outport
  wires:
  CMD_BRAKE_SP/1 -> Saturation/1
  PLA_SPEED_MS/1 -> Sign/1
  Sign/1 -> Product1/1
  Product1/1 -> Gain2/1
  Gain2/1 -> PLA_FORCE_BRAKE/1
  Saturation/1 -> Product1/2

== system AxleSplitHEVv6/HEV model/Platform/Mechanical behavior/Fengines ==
  PLA_TQ_SUM : Inport
  Gain1 : Gain  Gain=1/pla_wheel_radius  SampleTime=hev_dt
  PLA_FORCES_ENGINES : Outport
  wires:
  PLA_TQ_SUM/1 -> Gain1/1
  Gain1/1 -> PLA_FORCES_ENGINES/1

== system AxleSplitHEVv6/HEV model/Platform/Mechanical behavior/Ffriction ==
  PLA_SPEED_MS : Inport
  Abs : Abs  SampleTime=hev_dt
  Constant : Constant  Value=9.80665*pla_equivalent_weight*pla_f
  Constant2 : Constant  Value=9.80665*pla_equivalent_weight*pla_f*pla_csat
  Gain : Gain  Gain=-1  SampleTime=hev_dt
  Gain1 : Gain  Gain=pla_k*9.80665*pla_equivalent_weight  SampleTime=hev_dt
  Product : Product  SampleTime=hev_dt
  Sign : Signum  SampleTime=hev_dt
  Sum : Sum  Inputs=+|+  SampleTime=hev_dt
  Switch2 : Switch  Criteria=u2 > Threshold  Threshold=0.01  SampleTime=hev_dt
  PLA_FORCE_FRICTION : Outport
  wires:
  PLA_SPEED_MS/1 -> Abs/1, Sign/1  "v_m/s"
  Gain1/1 -> Sum/1
  Constant/1 -> Sum/2
  Abs/1 -> Gain1/1, Switch2/2
  Switch2/1 -> Product/1
  Product/1 -> Gain/1
  Sign/1 -> Product/2
  Gain/1 -> PLA_FORCE_FRICTION/1
  Sum/1 -> Switch2/1  "Froll"
  Constant2/1 -> Switch2/3

== system AxleSplitHEVv6/HEV model/Platform/Mechanical behavior/Fslope ==
  ENV_SLOPE_PERCENT : Inport
  PLA_SPEED_MS : Inport  Port=2
  Gain : Gain  Gain=-1  SampleTime=hev_dt
  Gain1 : Gain  Gain=0.01  SampleTime=hev_dt
  Gain2 : Gain  Gain=9.80665*pla_equivalent_weight  SampleTime=hev_dt
  Product : Product  SampleTime=hev_dt
  Product1 : Product  SampleTime=hev_dt
  Sign : Signum  SampleTime=hev_dt
  Sign1 : Signum  SampleTime=hev_dt
  Trigonometric Function : Trigonometry  Operator=atan  SampleTime=hev_dt
  Trigonometric Function1 : Trigonometry  SampleTime=hev_dt
  PLA_FORCE_SLOPE : Outport
  wires:
  ENV_SLOPE_PERCENT/1 -> Sign/1, Gain1/1
  Gain1/1 -> Trigonometric Function/1
  Trigonometric Function/1 -> Trigonometric Function1/1
  Trigonometric Function1/1 -> Gain2/1
  Gain/1 -> PLA_FORCE_SLOPE/1
  PLA_SPEED_MS/1 -> Sign1/1
  Sign/1 -> Product/1
  Sign1/1 -> Product/2
  Gain2/1 -> Product1/1
  Product/1 -> Product1/2
  Product1/1 -> Gain/1

== system AxleSplitHEVv6/HEV model/Rear Axle/Electrical machine/Engine representation ==
  CMD_RA_TQ_SP : Inport
  RA_N_EM : Inport  Port=2
  Discrete Transfer Fcn3 : DiscreteTransferFcn  Numerator=[(hev_dt/(2*(ra_electrical_machine_tau)+hev_dt)) (hev_dt/(2*(ra_electrical_machine_tau)+hev_dt))]  Denominator=[1 ((hev_dt-2*(ra_electrical_machine_tau)))/(2*(ra_electrical_machine_tau)+hev_dt)]  SampleTime=hev_dt
  Maximum torque : Lookup  InputValues=ra_electrical_machine_speed  Table=ra_em_max_tq  LookUpMeth=Interpolation-Use End Values  SampleTime=hev_dt
  Minimum torque : Lookup  InputValues=ra_electrical_machine_speed  Table=ra_em_min_tq  LookUpMeth=Interpolation-Use End Values  SampleTime=hev_dt
  Saturation Dynamic : simulink/Discontinuities/Saturation Dynamic  OutMin=[]  OutMax=[]  OutDataTypeStr=Inherit: Same as second input  OutDataType=fixdt(1, 16)  OutScaling=2^-10  DoSatur=off
  RA_TQ_ME : Outport
  RA_TQ_MIN_ME : Outport  Port=2
  RA_TQ_MAX_ME : Outport  Port=3
  wires:
  RA_N_EM/1 -> Maximum torque/1, Minimum torque/1
  Maximum torque/1 -> RA_TQ_MAX_ME/1, Saturation Dynamic/1
  Minimum torque/1 -> RA_TQ_MIN_ME/1, Saturation Dynamic/3
  Saturation Dynamic/1 -> Discrete Transfer Fcn3/1
  CMD_RA_TQ_SP/1 -> Saturation Dynamic/2
  Discrete Transfer Fcn3/1 -> RA_TQ_ME/1

== system AxleSplitHEVv6/HEV model/Rear Axle/Electrical machine/Power efficiency ==
  RA_TQ_ME : Inport
  RA_N_EM : Inport  Port=2
  Divide : Product  Inputs=/*  SampleTime=hev_dt
  Efficiency (%) : Lookup_n-D  BreakpointsForDimension1=ra_electrical_machine_torque  BreakpointsForDimension2=ra_electrical_machine_speed  Table=ra_electrical_machine_efficiency  SampleTime=hev_dt  RndMeth=Simplest  InputSameDT=on
  Efficiency conversion : Gain  Gain=1/100  SampleTime=hev_dt
  Product : Product  SampleTime=hev_dt  RndMeth=Zero
  Product1 : Product  SampleTime=hev_dt  RndMeth=Zero
  Switch : Switch  SampleTime=hev_dt
  "tr/min -> rad/s" : Gain  Gain=2*pi/60  SampleTime=hev_dt
  RA_EM_POWER : Outport
  wires:
  Efficiency (%)/1 -> Efficiency conversion/1
  Product/1 -> Switch/2, Product1/1, Divide/2
  Divide/1 -> Switch/1
  Product1/1 -> Switch/3
  Efficiency conversion/1 -> Product1/2, Divide/1
  "tr/min -> rad/s"/1 -> Product/2
  Switch/1 -> RA_EM_POWER/1  "W"
  RA_TQ_ME/1 -> Product/1, Efficiency (%)/1
  RA_N_EM/1 -> Efficiency (%)/2, "tr/min -> rad/s"/1

== system AxleSplitHEVv6/HEV model/Command/Torque repartition/Optimization Algorithm /Doc Front axle ==

== system AxleSplitHEVv6/HEV model/Command/Torque repartition/Optimization Algorithm /Doc Front axle1 ==

== system AxleSplitHEVv6/HEV model/Command/Torque repartition/Optimization Algorithm /Sfunction: Optimization Algorithm 32bits ==
  T : Inport
  V : Inport  Port=2
  Tmax_elec : Inport  Port=3
  Tmin_elec : Inport  Port=4
  Tmax_therm : Inport  Port=5
  Tmin_therm : Inport  Port=6
  GBX : Inport  Port=7
  SOC : Inport  Port=8
  MATLAB Function: Optimization Algorithm_sfcn : S-Function  FunctionName=MATLAB_sf  SFunctionModules=""  mask{rtw_sf_name=MATLAB_sf, showVar=off}
      mask prompts: rtw_sf_name "Simulink:masks:GenSFuncName_MP"; showVar "Simulink:masks:GenSFuncShowModuleList_MP"
      mask help: Simulink:masks:GenSFuncDesc_MD
      mask init:
      | displist = '';
      | if ~strcmp(get_param(gcb, 'FunctionName'), rtw_sf_name);
      |   set_param(gcb, 'FunctionName', rtw_sf_name);
      | end
      | % Check if we are generating code
      | rtw_mode = false;
      | if strcmpi(get_param(bdroot(gcb),'SimulationStatus'),'Initializing')
      | 	rtw_mode = strcmpi(get_param(bdroot(gcb),'BuildingRTWCode'),'on') && ...
      | 		~strcmpi(get_param(bdroot(gcb),'TargetStyle'),'SimulationTarget');
      | end
      | if showVar || rtw_mode
      | 	if exist('rtwsfunc') == 2 | exist('rtwsfunc') == 6
      | 		tmplist = rtwsfunc(rtw_sf_name,gcb);
      | 		tmplist = DAStudio.message('Simulink:masks:GenSFuncListOfModules_IC', tmplist);
      | 	elseif showVar
      | 		tmplist1 = DAStudio.message('Simulink:masks:GenSFuncListOfModules_IC', '');
      |         tmplist2 = DAStudio.message('Simulink:masks:GenSFuncNotLicensed_IC');
      |         tmplist = [tmplist1 tmplist2];
      |  	end
      | end
      | if showVar
      |   displist = tmplist;
      | end
      settings: CopyFcn=|
      | if ~strcmp(get_param(gcb,'Linkstatus'),'none') && ...
      | ~strcmp(get_param(gcb,'Linkstatus'),'implicit')
      |   set_param(gcb,'LinkStatus','none');
      | end
      mask Help: eval('feval(''rtwprivate'',''rtwhelpview'',''rtw_sfcn_block'')');
      mask Display:
      | port_label('input',1,'T');
      | port_label('input',2,'V');
      | port_label('input',3,'Tmax_elec');
      | port_label('input',4,'Tmin_elec');
      | port_label('input',5,'Tmax_therm');
      | port_label('input',6,'Tmin_therm');
      | port_label('input',7,'GBX');
      | port_label('input',8,'SOC');
      | port_label('output',1,'alpha_opt');
  __InputSSForSFun__ : Subsystem
  __OutputSSForSFun__ : Subsystem
  alpha_opt : Outport
  wires:
  T/1 -> __InputSSForSFun__/1(T)
  V/1 -> __InputSSForSFun__/2(V)
  Tmax_elec/1 -> __InputSSForSFun__/3(Tmax_elec)
  Tmin_elec/1 -> __InputSSForSFun__/4(Tmin_elec)
  Tmax_therm/1 -> __InputSSForSFun__/5(Tmax_therm)
  Tmin_therm/1 -> __InputSSForSFun__/6(Tmin_therm)
  GBX/1 -> __InputSSForSFun__/7(GBX)
  SOC/1 -> __InputSSForSFun__/8(SOC)
  __InputSSForSFun__/1(__UniqueOutportName__1__) -> MATLAB Function: Optimization Algorithm_sfcn/1
  __InputSSForSFun__/2(__UniqueOutportName__2__) -> MATLAB Function: Optimization Algorithm_sfcn/2
  __InputSSForSFun__/3(__UniqueOutportName__3__) -> MATLAB Function: Optimization Algorithm_sfcn/3
  __InputSSForSFun__/4(__UniqueOutportName__4__) -> MATLAB Function: Optimization Algorithm_sfcn/4
  __InputSSForSFun__/5(__UniqueOutportName__5__) -> MATLAB Function: Optimization Algorithm_sfcn/5
  __InputSSForSFun__/6(__UniqueOutportName__6__) -> MATLAB Function: Optimization Algorithm_sfcn/6
  __InputSSForSFun__/7(__UniqueOutportName__7__) -> MATLAB Function: Optimization Algorithm_sfcn/7
  __InputSSForSFun__/8(__UniqueOutportName__8__) -> MATLAB Function: Optimization Algorithm_sfcn/8
  MATLAB Function: Optimization Algorithm_sfcn/1 -> __OutputSSForSFun__/1(__UniqueInportName__1__)
  __OutputSSForSFun__/1(alpha_opt) -> alpha_opt/1

== system AxleSplitHEVv6/HEV model/Electrical system/Lithium-Ion Battery Management System/Battery model/li-ion Battery SOC ==
  SYSE_LIION_CURRENT : Inport
  Discrete-Time Integrator : DiscreteIntegrator  IntegratorMethod=Integration: Trapezoidal  InitialConditionSource=external  SampleTime=hev_dt  LimitOutput=on  UpperSaturationLimit=1  LowerSaturationLimit=0
  Divide1 : Product  Inputs=/*  SampleTime=hev_dt
  Gain : Gain  Gain=-1  SampleTime=hev_dt
  Nominal capacity : Constant  Value=syse_bat_nominal_capacity_as
  syse_soc_initial : Constant  Value=syse_soc_initial
  SYSE_SOC : Outport
  wires:
  Nominal capacity/1 -> Divide1/1  "A.s"
  Discrete-Time Integrator/1 -> SYSE_SOC/1
  syse_soc_initial/1 -> Discrete-Time Integrator/2
  Divide1/1 -> Discrete-Time Integrator/1  "s"
  SYSE_LIION_CURRENT/1 -> Gain/1  "A"
  Gain/1 -> Divide1/2

== system AxleSplitHEVv6/HEV model/Electrical system/Lithium-Ion Battery Management System/Battery model/li-ion battery voltage ==
  SYSE_SOC : Inport
  SYSE_LIION_CURRENT : Inport  Port=2
  Add2 : Sum  Inputs=+--  SampleTime=hev_dt
  Discrete Transfer Fcn1 : DiscreteTransferFcn  Numerator=[(hev_dt/(2*(syse_rdl*syse_cdl)+hev_dt)) (hev_dt/(2* (syse_rdl*syse_cdl)+hev_dt))]  Denominator=[1 ((hev_dt-2*(syse_rdl*syse_cdl)))/(2*(syse_rdl*syse_cdl)+hev_dt)]  SampleTime=hev_dt
  Gain : Gain  Gain=syse_rdl  SampleTime=hev_dt
  Lookup table Vocv : Lookup_n-D  NumberOfTableDimensions=1  BreakpointsForDimension1=syse_soc_ocv/100  Table=syse_vocv  SampleTime=hev_dt  RndMeth=Simplest  InputSameDT=on
  Rser : Gain  Gain=syse_rser  SampleTime=hev_dt
  nb of cell : Gain  Gain=syse_nb_cell  SampleTime=hev_dt
  SYSE_VOLTAGE_HV : Outport
  wires:
  SYSE_LIION_CURRENT/1 -> Gain/1, Rser/1
  SYSE_SOC/1 -> Lookup table Vocv/1
  Lookup table Vocv/1 -> Add2/1
  Add2/1 -> nb of cell/1
  nb of cell/1 -> SYSE_VOLTAGE_HV/1
  Rser/1 -> Add2/2
  Discrete Transfer Fcn1/1 -> Add2/3
  Gain/1 -> Discrete Transfer Fcn1/1

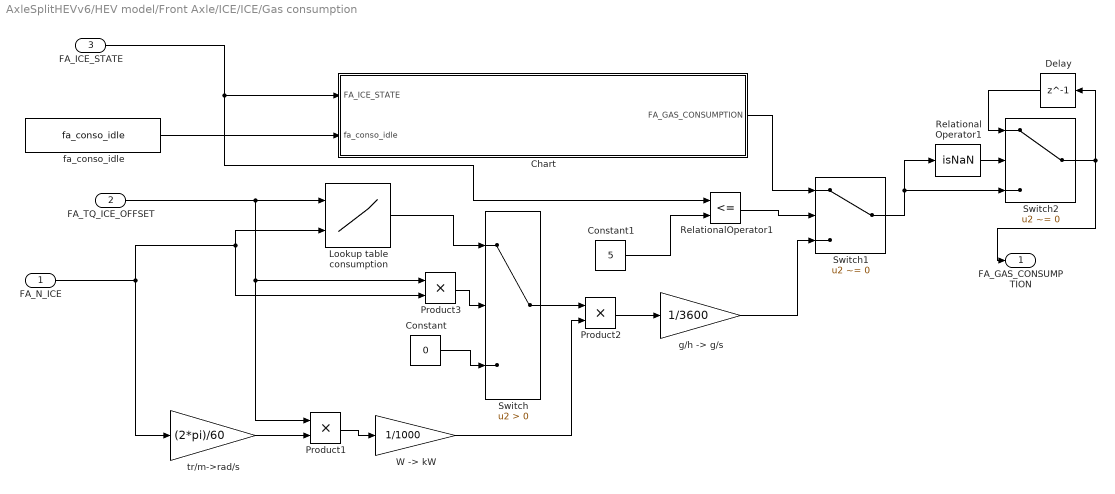
== system AxleSplitHEVv6/HEV model/Front Axle/ICE/ICE/Gas consumption ==
  FA_N_ICE : Inport
  FA_TQ_ICE_OFFSET : Inport  Port=2
  FA_ICE_STATE : Inport  Port=3
  Chart : Stateflow chart  TreatAsAtomicUnit=on
  Constant : Constant  Value=0
  Constant1 : Constant  Value=5
  Delay : Delay  DelayLength=1  SampleTime=hev_dt
  Lookup table consumption : Lookup_n-D  BreakpointsForDimension1=fa_conso_torque  BreakpointsForDimension2=fa_conso_speed  Table=fa_fuel_consumption  ExtrapMethod=Clip  UseLastTableValue=on  SampleTime=hev_dt  RndMeth=Simplest  InputSameDT=on
  Product1 : Product  SampleTime=hev_dt  RndMeth=Zero
  Product2 : Product  SampleTime=hev_dt  RndMeth=Zero
  Product3 : Product  SampleTime=hev_dt  RndMeth=Zero
  Relational Operator1 : RelationalOperator  Operator=isNaN  OutDataTypeStr=boolean  SampleTime=hev_dt
  RelationalOperator1 : RelationalOperator  Operator=<=  OutDataTypeStr=boolean  SampleTime=hev_dt
  Switch : Switch  Criteria=u2 > Threshold  SampleTime=hev_dt
  Switch1 : Switch  Criteria=u2 ~= 0  SampleTime=hev_dt
  Switch2 : Switch  Criteria=u2 ~= 0  SampleTime=hev_dt
  "W -> kW" : Gain  Gain=1/1000  SampleTime=hev_dt
  fa_conso_idle : Constant  Value=fa_conso_idle
  "g/h -> g/s" : Gain  Gain=1/3600  SampleTime=hev_dt
  tr/m->rad/s : Gain  Gain=(2*pi)/60  SampleTime=hev_dt
  FA_GAS_CONSUMPTION : Outport
  wires:
  Lookup table consumption/1 -> Switch/1
  Switch/1 -> Product2/1
  Constant/1 -> Switch/3
  "W -> kW"/1 -> Product2/2
  Product1/1 -> "W -> kW"/1
  tr/m->rad/s/1 -> Product1/2
  Product2/1 -> "g/h -> g/s"/1
  FA_N_ICE/1 -> Lookup table consumption/2, Product3/2, tr/m->rad/s/1
  FA_TQ_ICE_OFFSET/1 -> Product3/1, Product1/1, Lookup table consumption/1
  Product3/1 -> Switch/2
  Switch1/1 -> Switch2/3, Relational Operator1/1
  Switch2/1 -> FA_GAS_CONSUMPTION/1, Delay/1
  Relational Operator1/1 -> Switch2/2
  Delay/1 -> Switch2/1
  FA_ICE_STATE/1 -> RelationalOperator1/1, Chart/1(FA_ICE_STATE)
  "g/h -> g/s"/1 -> Switch1/3
  Chart/1(FA_GAS_CONSUMPTION) -> Switch1/1
  Constant1/1 -> RelationalOperator1/2
  RelationalOperator1/1 -> Switch1/2
  fa_conso_idle/1 -> Chart/2(fa_conso_idle)

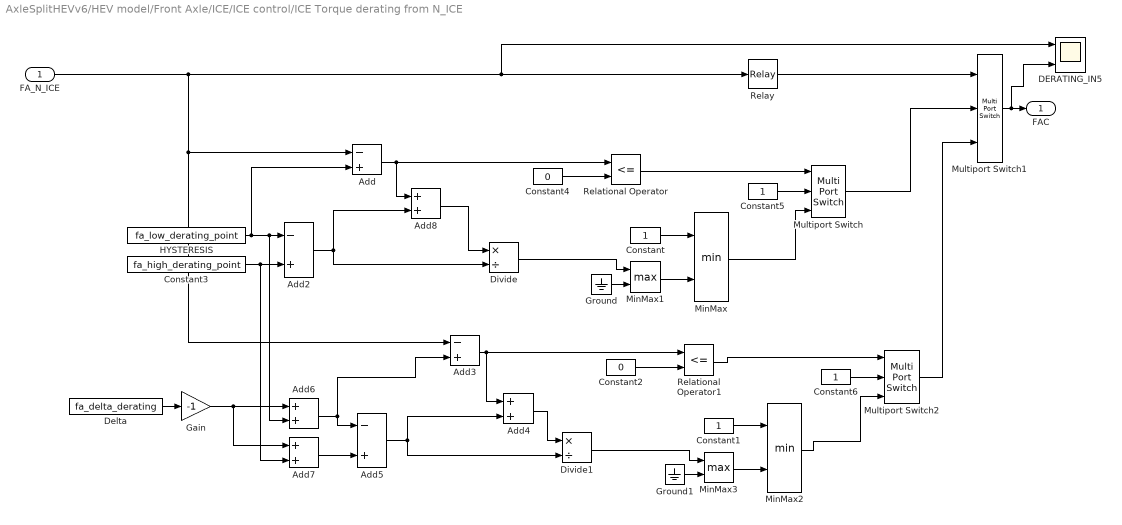
== system AxleSplitHEVv6/HEV model/Front Axle/ICE/ICE control/ICE Torque derating from N_ICE ==
  FA_N_ICE : Inport
  Add{,2..3,5} (4 alike) : Sum  Inputs=-+
  Add{4,6..8} (4 alike) : Sum
  Constant{,1,5..6} (4 alike) : Constant
  Constant2 : Constant  Value=0
  Constant3 : Constant  Value=fa_high_derating_point
  Constant4 : Constant  Value=0
  DERATING_IN5 : Scope  NumInputPorts=2
      settings: ShowLegends=on  TimeRange=1180  YMin=0~-0.5  YMax=6000~1.5  SaveName=ScopeData23
  Delta : Constant  Value=fa_delta_derating
  Divide : Product  Inputs=*/
  Divide1 : Product  Inputs=*/
  Gain : Gain  Gain=-1
  Ground : Ground
  Ground1 : Ground
  HYSTERESIS : Constant  Value=fa_low_derating_point
  MinMax : MinMax  Inputs=2
  MinMax1 : MinMax  Function=max  Inputs=2
  MinMax2 : MinMax  Inputs=2
  MinMax3 : MinMax  Function=max  Inputs=2
  Multiport Switch : MultiPortSwitch  DataPortOrder=Zero-based contiguous  Inputs=2
  Multiport Switch1 : MultiPortSwitch  DataPortOrder=Zero-based contiguous  Inputs=2
  Multiport Switch2 : MultiPortSwitch  DataPortOrder=Zero-based contiguous  Inputs=2
  Relational Operator : RelationalOperator  Operator=<=  OutDataTypeStr=boolean
  Relational Operator1 : RelationalOperator  Operator=<=  OutDataTypeStr=boolean
  Relay : Relay  OnSwitchValue=5750  OffSwitchValue=4900-500
  FAC : Outport
  wires:
  Gain/1 -> Add6/1, Add7/1
  Add4/1 -> Divide1/1
  Add8/1 -> Divide/1
  Add7/1 -> Add5/2
  Add6/1 -> Add3/2, Add5/1
  Constant6/1 -> Multiport Switch2/2
  MinMax2/1 -> Multiport Switch2/3
  Relational Operator1/1 -> Multiport Switch2/1
  Constant2/1 -> Relational Operator1/2
  Add3/1 -> Relational Operator1/1, Add4/1
  Divide1/1 -> MinMax3/1
  MinMax3/1 -> MinMax2/2
  Ground1/1 -> MinMax3/2
  Constant1/1 -> MinMax2/1
  FA_N_ICE/1 -> Add3/1, Add/1, Relay/1, DERATING_IN5/1
  Delta/1 -> Gain/1
  Constant3/1 -> Add2/2, Add7/2
  Multiport Switch2/1 -> Multiport Switch1/3
  HYSTERESIS/1 -> Add6/2, Add2/1, Add/2
  Multiport Switch/1 -> Multiport Switch1/2
  Constant5/1 -> Multiport Switch/2
  MinMax/1 -> Multiport Switch/3
  Relational Operator/1 -> Multiport Switch/1
  Constant4/1 -> Relational Operator/2
  Add/1 -> Add8/1, Relational Operator/1
  Relay/1 -> Multiport Switch1/1
  Divide/1 -> MinMax1/1
  MinMax1/1 -> MinMax/2
  Ground/1 -> MinMax1/2
  Constant/1 -> MinMax/1
  Multiport Switch1/1 -> FAC/1, DERATING_IN5/2
  Add2/1 -> Divide/2, Add8/2
  Add5/1 -> Divide1/2, Add4/2
